simulink model "Encoder_reading"  (R2024b)
settings: Solver=FixedStepAuto  StartTime=0.0  StopTime=inf  FixedStep=0.01  RelTol=1e-3  EnableMultiTasking=on
libraries: stm32f4xxblockslib x3, stm32g4xxblockslib x3
settings Model: STM32="{\"EncoderBlockForG4\":[{\"ID\":\"untitled:1\"},{\"ID\":\"untitled:4\"},{\"ID\":\"untitled:5\"},{\"ID\":\"Encoder_reading:1\"},{\"ID\":\"Encoder_reading:4\"},{\"ID\":\"Encoder_reading:5\"}],\"DigitalPortRead\":[{\"ID\":\"untitled:12\"},{\"ID\":\"untitled:16\"},{\"ID\":\"untitled:17\"},{\"ID\":\"untitled:18\"},{\"ID\":\"untitled:19\"},{\"ID\":\"untitled:20\"},{\"ID\":\"Encoder_reading:16\"},{\"ID\":\"Encoder_reading:12\"},{\"ID\":\"Encoder_reading:147\"}]}"  Creator=Kaitniyom  LastModifiedBy=Kaitniyom
settings OptimizationCC: DefaultParameterBehavior=Inlined  EnhancedBackFolding=on  PassReuseOutputArgsAs=Individual arguments  ZeroExternalMemoryAtStartup=off  ZeroInternalMemoryAtStartup=off  MaxStackSize=512  OptimizeBlockOrder=speed  DifferentSizesBufferReuse=on  OptimizationCustomize=off  EfficientTunableParamExpr=on
settings DebuggingCC: ParameterTunabilityLossMsg=error
settings HardwareCC: ProdBitPerPointer=32  ProdBitPerSizeT=32  ProdBitPerPtrDiffT=32  ProdLargestAtomicInteger=Long  ProdLargestAtomicFloat=Double  ProdWordSize=32  ProdLongLongMode=on  ProdHWDeviceType=ARM Compatible->ARM Cortex-M
settings SFSimCC: MATLABDynamicMemAlloc=off
settings RTWCC: Description=Embedded Coder  SystemTargetFile=ert.tlc  HardwareBoard=STM32G4xx Based  TemplateMakefile=ert_default_tmf  Toolchain=GNU Tools for ARM Embedded Processors
settings CodeAppCC: ForceParamTrailComments=on  IgnoreCustomStorageClasses=off  OperatorAnnotations=on  SimulinkDataObjDesc=on  SFDataObjDesc=on  InsertBlockDesc=on
settings ERTTargetCC: TargetLangStandard=C99 (ISO)  CodeReplacementLibrary=ARM Cortex-M  SupportContinuousTime=on  ExtModeTransport=3  ExtModeStaticAlloc=on  ExtModeStaticAllocSize=2048  ExtModeMexFile=ext_xcp  ExtModeIntrfLevel=Level2 - Open

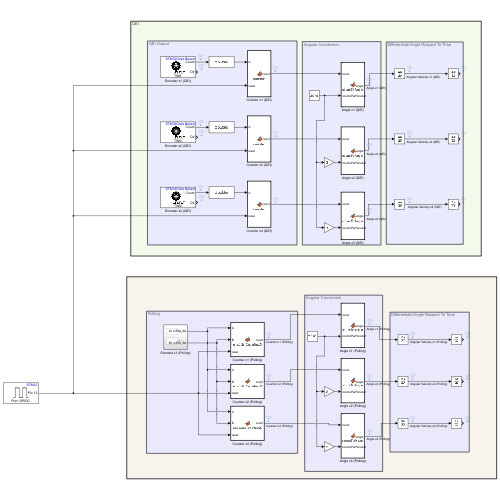
[thumbnail: Simulink's stored preview of the top-level diagram]
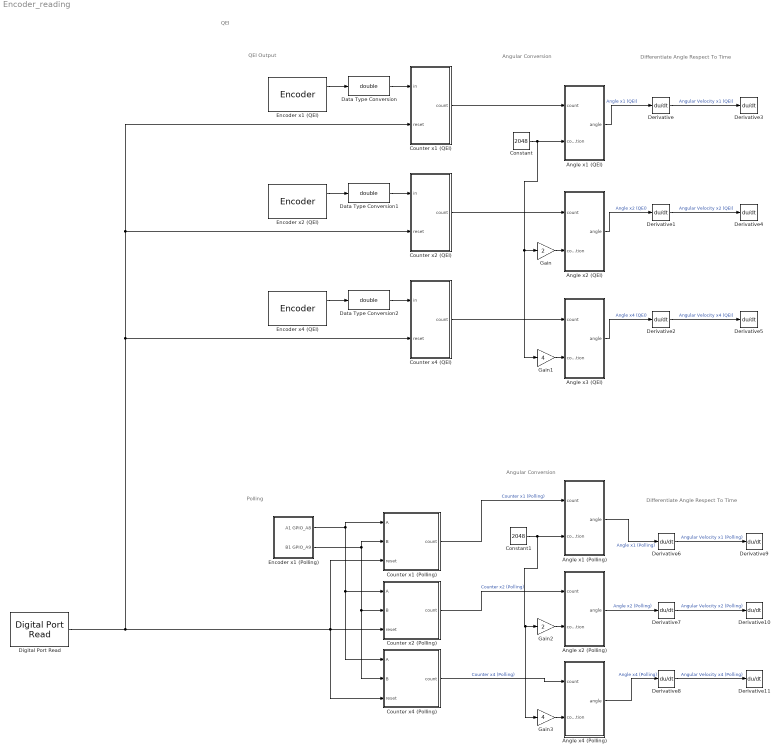
== system Encoder_reading ==
  note: QEI
  note: Angular Conversion
  note: Differentiate Angle Respect To Time
  note: Polling
  note: Differentiate Angle Respect To Time
  note: Angular Conversion
  note: QEI Output
  Angle x1 (Polling) : MATLAB Function  TreatAsAtomicUnit=on
  Angle x1 (QEI) : MATLAB Function  TreatAsAtomicUnit=on
  Angle x2 (Polling) : MATLAB Function  TreatAsAtomicUnit=on
  Angle x2 (QEI) : MATLAB Function  TreatAsAtomicUnit=on
  Angle x3 (QEI) : MATLAB Function  TreatAsAtomicUnit=on
  Angle x4 (Polling) : MATLAB Function  TreatAsAtomicUnit=on
  Constant : Constant  Value=2048
  Constant1 : Constant  Value=2048
  Counter x1 (Polling) : MATLAB Function  TreatAsAtomicUnit=on
  Counter x1 (QEI) : MATLAB Function  TreatAsAtomicUnit=on
  Counter x2 (Polling) : MATLAB Function  TreatAsAtomicUnit=on
  Counter x2 (QEI) : MATLAB Function  TreatAsAtomicUnit=on
  Counter x4 (Polling) : MATLAB Function  TreatAsAtomicUnit=on
  Counter x4 (QEI) : MATLAB Function  TreatAsAtomicUnit=on
  Data Type Conversion : DataTypeConversion  OutDataTypeStr=double  SaturateOnIntegerOverflow=off  RndMeth=Floor
  Data Type Conversion1 : DataTypeConversion  OutDataTypeStr=double  SaturateOnIntegerOverflow=off  RndMeth=Floor
  Data Type Conversion2 : DataTypeConversion  OutDataTypeStr=double  SaturateOnIntegerOverflow=off  RndMeth=Floor
  Derivative{,1..11} (12 alike) : Derivative
  Digital Port Read : stm32f4xxblockslib/Digital Port Read  PortName=GPIOC  PinNumber=13  ReadOperation=on  IOAsArray=off  SampleTime=-1  EnableSimPort=off  hoistedMaskSrc=ECSoC/ECSimCodegen/Digital Port Read
      settings: LibrarySourceBlock=stm32g4xxblockslib/Digital Port Read
  Encoder x1 (Polling) : Subsystem
  Encoder x1 (QEI) : stm32g4xxblockslib/Encoder  TimerModule=TIM1  EnableResetInput=off  OutputCountAfterFirstIndex=off  OutputValidIndex=off  OutputDirection=on  OutputStatus=off  SampleTime=-1
  Encoder x2 (QEI) : stm32g4xxblockslib/Encoder  TimerModule=TIM3  EnableResetInput=off  OutputCountAfterFirstIndex=off  OutputValidIndex=off  OutputDirection=on  OutputStatus=off  SampleTime=-1
  Encoder x4 (QEI) : stm32g4xxblockslib/Encoder  TimerModule=TIM4  EnableResetInput=off  OutputCountAfterFirstIndex=off  OutputValidIndex=off  OutputDirection=on  OutputStatus=off  SampleTime=-1
  Gain : Gain  Gain=2
  Gain1 : Gain  Gain=4
  Gain2 : Gain  Gain=2
  Gain3 : Gain  Gain=4
  wires:
  Data Type Conversion/1 -> Counter x1 (QEI)/1(in)
  Encoder x2 (QEI)/1 -> Data Type Conversion1/1
  Encoder x4 (QEI)/1 -> Data Type Conversion2/1
  Encoder x1 (QEI)/1 -> Data Type Conversion/1
  Data Type Conversion1/1 -> Counter x2 (QEI)/1(in)
  Data Type Conversion2/1 -> Counter x4 (QEI)/1(in)
  Counter x1 (QEI)/1(count) -> Angle x1 (QEI)/1(count)
  Counter x2 (QEI)/1(count) -> Angle x2 (QEI)/1(count)
  Counter x4 (QEI)/1(count) -> Angle x3 (QEI)/1(count)
  Angle x1 (QEI)/1(angle) -> Derivative/1  "Angle x1 (QEI)"
  Angle x2 (QEI)/1(angle) -> Derivative1/1  "Angle x2 (QEI)"
  Angle x3 (QEI)/1(angle) -> Derivative2/1  "Angle x4 (QEI)"
  Derivative/1 -> Derivative3/1  "Angular Velocity x1 (QEI)"
  Derivative1/1 -> Derivative4/1  "Angular Velocity x2 (QEI)"
  Derivative2/1 -> Derivative5/1  "Angular Velocity x4 (QEI)"
  Counter x1 (Polling)/1(count) -> Angle x1 (Polling)/1(count)  "Counter x1 (Polling)"
  Counter x2 (Polling)/1(count) -> Angle x2 (Polling)/1(count)  "Counter x2 (Polling)"
  Counter x4 (Polling)/1(count) -> Angle x4 (Polling)/1(count)  "Counter x4 (Polling)"
  Derivative6/1 -> Derivative9/1  "Angular Velocity x1 (Polling)"
  Derivative7/1 -> Derivative10/1  "Angular Velocity x2 (Polling)"
  Derivative8/1 -> Derivative11/1  "Angular Velocity x4 (Polling)"
  Encoder x1 (Polling)/1(A1 GPIO_A8) -> Counter x1 (Polling)/1(A), Counter x4 (Polling)/1(A), Counter x2 (Polling)/1(A)
  Encoder x1 (Polling)/2(B1 GPIO_A9) -> Counter x4 (Polling)/2(B), Counter x2 (Polling)/2(B), Counter x1 (Polling)/2(B)
  Gain/1 -> Angle x2 (QEI)/2(countsPerRevolution)
  Gain1/1 -> Angle x3 (QEI)/2(countsPerRevolution)
  Gain2/1 -> Angle x2 (Polling)/2(countsPerRevolution)
  Gain3/1 -> Angle x4 (Polling)/2(countsPerRevolution)
  Constant/1 -> Gain1/1, Gain/1, Angle x1 (QEI)/2(countsPerRevolution)
  Angle x1 (Polling)/1(angle) -> Derivative6/1  "Angle x1 (Polling)"
  Angle x2 (Polling)/1(angle) -> Derivative7/1  "Angle x2 (Polling)"
  Angle x4 (Polling)/1(angle) -> Derivative8/1  "Angle x4 (Polling)"
  Constant1/1 -> Gain3/1, Gain2/1, Angle x1 (Polling)/2(countsPerRevolution)
  Digital Port Read/1 -> Counter x2 (QEI)/2(reset), Counter x1 (QEI)/2(reset), Counter x4 (QEI)/2(reset), Counter x1 (Polling)/3(reset), Counter x2 (Polling)/3(reset), Counter x4 (Polling)/3(reset)

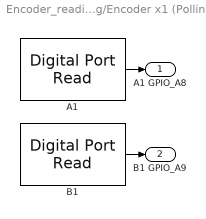
== system Encoder_reading/Encoder x1 (Polling) ==
  A1 : stm32f4xxblockslib/Digital Port Read  PortName=GPIOA  PinNumber=8  ReadOperation=on  IOAsArray=off  SampleTime=-1  EnableSimPort=off  hoistedMaskSrc=ECSoC/ECSimCodegen/Digital Port Read
      settings: LibrarySourceBlock=stm32g4xxblockslib/Digital Port Read
  B1 : stm32f4xxblockslib/Digital Port Read  PortName=GPIOA  PinNumber=9  ReadOperation=on  IOAsArray=off  SampleTime=-1  EnableSimPort=off  hoistedMaskSrc=ECSoC/ECSimCodegen/Digital Port Read
      settings: LibrarySourceBlock=stm32g4xxblockslib/Digital Port Read
  A1 GPIO_A8 : Outport
  B1 GPIO_A9 : Outport  Port=2
  wires:
  B1/1 -> B1 GPIO_A9/1
  A1/1 -> A1 GPIO_A8/1

== matlab function Encoder_reading/Angle x4 (Polling) ==
  data: count input; angle output; countsPerRevolution input
function angle = countToAngle(count, countsPerRevolution)
    % countToAngle converts encoder count to an angle in radians
    
    % Calculate angle in radians
    angle = (count / countsPerRevolution) * 2 * pi;
end

== matlab function Encoder_reading/Counter x1 (QEI) ==
  data: in input; count output; reset input
function count = counter(in, reset)
    persistent i prev;
    count_period = 65520;  % Set count_period 

    if isempty(i)  
        i = 0;  
        prev = 0;       
    end

    if reset == 1
        i = 0;
    end

    % Calculate the difference between the current and previous encoder position
    diff = in - prev;

    % Define a threshold for detecting wrap-around (half of count_period)
    threshold = count_period / 2;

    % Adjust i based on diff, accounting for adaptive wrap-around detection
    if diff > threshold       % Wrapped forward (overflow)
        i = i - (count_period - diff) - 1;
    elseif diff < -threshold  % Wrapped backward (underflow)
        i = i + (count_period + diff) + 1;
    else
        i = i + diff;         % Normal increment or decrement
    end

    % Update previous value for the next iteration
    prev = in;
    count = i;
end

== matlab function Encoder_reading/Counter x2 (QEI) ==
  data: in input; count output; reset input
function count = counter(in, reset)
    persistent i prev;
    count_period = 65520;  % Set count_period directly in the function

    if isempty(i)  
        i = 0;  
        prev = 0;       
    end
    
    if reset == 1
        i = 0;
    end

    % Calculate the difference between the current and previous encoder position
    diff = in - prev;

    % Define a threshold for detecting wrap-around (half of count_period)
    threshold = count_period / 2;

    % Adjust i based on diff, accounting for adaptive wrap-around detection
    if diff > threshold       % Wrapped forward (overflow)
        i = i - (count_period - diff) - 1;
    elseif diff < -threshold  % Wrapped backward (underflow)
        i = i + (count_period + diff) + 1;
    else
        i = i + diff;         % Normal increment or decrement
    end

    % Update previous value for the next iteration
    prev = in;
    count = i;
end

== matlab function Encoder_reading/Counter x4 (QEI) ==
  data: in input; count output; reset input
function count = counter(in, reset)
    persistent i prev;
    count_period = 65472;  % Set count_period directly in the function

    if isempty(i)  
        i = 0;  
        prev = 0;       
    end

    if reset == 1
        i = 0;
    end

    % Calculate the difference between the current and previous encoder position
    diff = in - prev;

    % Define a threshold for detecting wrap-around (half of count_period)
    threshold = count_period / 2;

    % Adjust i based on diff, accounting for adaptive wrap-around detection
    if diff > threshold       % Wrapped forward (overflow)
        i = i - (count_period - diff) - 1;
    elseif diff < -threshold  % Wrapped backward (underflow)
        i = i + (count_period + diff) + 1;
    else
        i = i + diff;         % Normal increment or decrement
    end

    % Update previous value for the next iteration
    prev = in;
    count = i;
end

== matlab function Encoder_reading/Angle x1 (QEI) ==
  data: count input; angle output; countsPerRevolution input
function angle = countToAngle(count, countsPerRevolution)
    % countToAngle converts encoder count to an angle in radians
    
    % Calculate angle in radians
    angle = (count / countsPerRevolution) * 2 * pi;
end

== matlab function Encoder_reading/Angle x2 (QEI) ==
  data: count input; angle output; countsPerRevolution input
function angle = countToAngle(count, countsPerRevolution)
    % countToAngle converts encoder count to an angle in radians
    
    % Calculate angle in radians
    angle = (count / countsPerRevolution) * 2 * pi;
end

== matlab function Encoder_reading/Angle x3 (QEI) ==
  data: count input; angle output; countsPerRevolution input
function angle = countToAngle(count, countsPerRevolution)
    % countToAngle converts encoder count to an angle in radians
    
    % Calculate angle in radians
    angle = (count / countsPerRevolution) * 2 * pi;
end

== matlab function Encoder_reading/Counter x2 (Polling) ==
  data: A input; count output; B input; reset input
function count = encoderCounterx2(A, B, reset)
    persistent lastA i;
    if isempty(lastA)
        lastA = false;
        i = 0;  % Encoder count
    end

    if reset == 1
        i = 0;
    end

    % Check for a change in A (rising or falling edge)
    if A ~= lastA
        if A == true  % Rising edge
            if B == false
                i = i + 1;
            else
                i = i - 1;
            end
        else  % Falling edge
            if B == true
                i = i + 1;
            else
                i = i - 1;
            end
        end
    end

    lastA = A;  % Update lastA for next edge detection
    count = i;
end

== matlab function Encoder_reading/Counter x4 (Polling) ==
  data: A input; count output; B input; reset input
function count = encoderCounterx4(A, B, reset)
    persistent lastA lastB i;
    if isempty(lastA)
        lastA = false;
        lastB = false;
        i = 0;  % Encoder count
    end
    
    if reset == 1
        i = 0;
    end

    % Check for a change in either A or B
    if A ~= lastA || B ~= lastB
        % Determine direction based on transitions in A and B
        if lastA == false && A == true  % Rising edge on A
            if B == false
                i = i + 1;
            else
                i = i - 1;
            end
        elseif lastA == true && A == false  % Falling edge on A
            if B == true
                i = i + 1;
            else
                i = i - 1;
            end
        elseif lastB == false && B == true  % Rising edge on B
            if A == true
                i = i + 1;
            else
                i = i - 1;
            end
        elseif lastB == true && B == false  % Falling edge on B
            if A == false
                i = i + 1;
            else
                i = i - 1;
            end
        end
    end

    % Update lastA and lastB for next edge detection
    lastA = A;
    lastB = B;
    count = i;
end

== matlab function Encoder_reading/Angle x1 (Polling) ==
  data: count input; angle output; countsPerRevolution input
function angle = countToAngle(count, countsPerRevolution)
    % countToAngle converts encoder count to an angle in radians
    
    % Calculate angle in radians
    angle = (count / countsPerRevolution) * 2 * pi;
end

== matlab function Encoder_reading/Counter x1 (Polling) ==
  data: A input; count output; B input; reset input
function count = encoderCounterx1(A, B, reset)
    persistent lastA i;
    if isempty(lastA)
        lastA = false;
        i = 0;  % Encoder count
    end

    if reset == 1
        i = 0;
    end

    if A ~= lastA  % Detect change in A to indicate an edge
        if A == true && B == false
            i = i + 1;  % Increment
        elseif A == true && B == true
            i = i - 1;  % Decrement
        end
    end

    lastA = A;  % Update lastA for next edge detection
    count = i;
end

== matlab function Encoder_reading/Angle x2 (Polling) ==
  data: count input; angle output; countsPerRevolution input
function angle = countToAngle(count, countsPerRevolution)
    % countToAngle converts encoder count to an angle in radians
    
    % Calculate angle in radians
    angle = (count / countsPerRevolution) * 2 * pi;
end
